simulink model "DC_control"  (R2023b)
settings: configuration reference "ctrl_tsk_conf" (kept outside this file)
settings Model: DataDictionary=fmuGenerationDictionay.sldd  ModifiedByFormat=Third Equation Ltd  Creator=Third Equation Ltd  LastModifiedBy=Third Equation Ltd
settings ConfigSetRef: SourceName=ctrl_tsk_conf

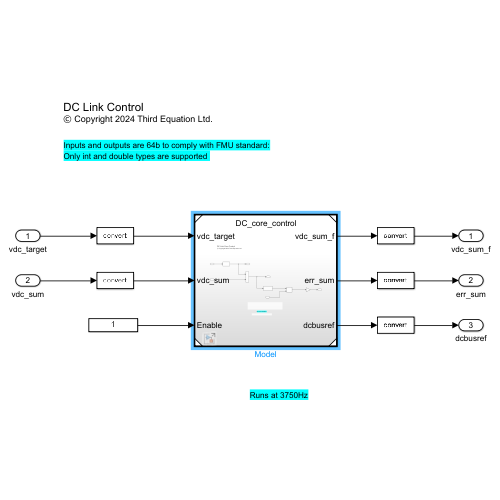
[thumbnail: Simulink's stored preview of the top-level diagram]
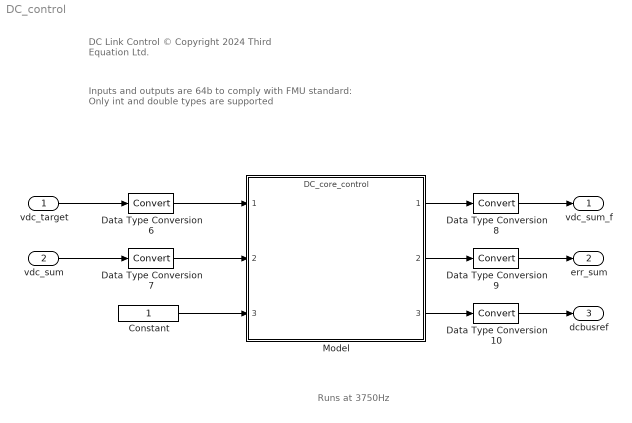
== system DC_control ==
  note: Inputs and outputs are 64b to comply with FMU standard:
      | Only int and double types are supported
  note: DC Link Control
      | © Copyright 2024 Third Equation Ltd.
  note: Runs at 3750Hz
  vdc_target : Inport
  vdc_sum : Inport  Port=2
  Constant : Constant  OutDataTypeStr=Inherit: Inherit via back propagation
  Data Type Conversion{6..10} (5 alike) : DataTypeConversion  SaturateOnIntegerOverflow=off  RndMeth=Floor
  Model : ModelReference  ModelNameDialog=DC_core_control.slx  SimulationMode=Normal  ModelReferenceVersion=1.22
  vdc_sum_f : Outport  OutDataTypeStr=double
  err_sum : Outport  Port=2  OutDataTypeStr=double
  dcbusref : Outport  Port=3  OutDataTypeStr=double
  wires:
  Constant/1 -> Model/3
  Data Type Conversion6/1 -> Model/1
  vdc_target/1 -> Data Type Conversion6/1
  Data Type Conversion7/1 -> Model/2
  vdc_sum/1 -> Data Type Conversion7/1
  Model/1 -> Data Type Conversion8/1
  Model/2 -> Data Type Conversion9/1
  Model/3 -> Data Type Conversion10/1
  Data Type Conversion8/1 -> vdc_sum_f/1
  Data Type Conversion9/1 -> err_sum/1
  Data Type Conversion10/1 -> dcbusref/1
